simulink subsystem "Magnetometer"  (R2021a)
settings: Solver=VariableStepAuto  StartTime=0.0  StopTime=10.0  RelTol=1e-3
libraries: simulink x4, sharedtransform x1
settings Model: Creator=jmher  LastModifiedBy=jmher

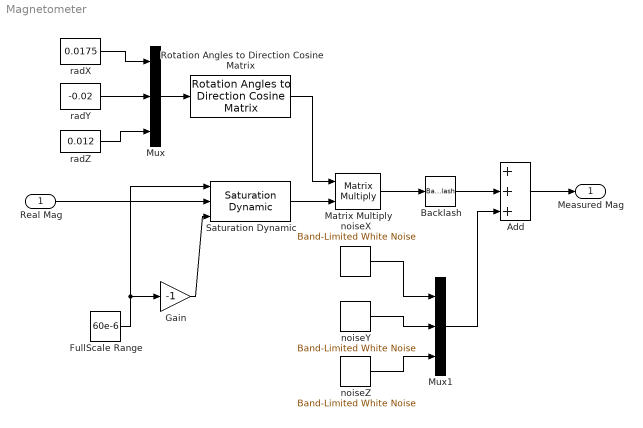
== system Magnetometer ==
  Real Mag : Inport
  Add : Sum  Inputs=+|+|+
  Backlash : Backlash  BacklashWidth=hyst  InputProcessing=Columns as channels (frame based)
  FullScale Range : Constant  Value=60e-6
  Gain : Gain  Gain=-1
  Matrix Multiply : Product  Multiplication=Matrix(*)
  Mux : Mux  Inputs=3
  Mux1 : Mux  Inputs=3
  Rotation Angles to Direction Cosine Matrix : sharedtransform/Rotation Angles to Direction Cosine Matrix  rotationOrder=ZYX  aMode=aMode
      settings: SourceProductBaseCode=AE,PW,DR,MT,UV,VE
  Saturation Dynamic : simulink/Discontinuities/Saturation Dynamic  OutMin=[]  OutMax=[]  OutDataTypeStr=Inherit: Same as second input  OutDataType=fixdt(1, 16)  OutScaling=2^-10  DoSatur=off
  noiseX : simulink/Sources/Band-Limited White Noise  Cov=noiseDens  Ts=0.1  seed=[47561]
  noiseY : simulink/Sources/Band-Limited White Noise  Cov=noiseDens  Ts=0.1  seed=[238641]
  noiseZ : simulink/Sources/Band-Limited White Noise  Cov=noiseDens  Ts=0.1  seed=[23341]
  radX : Constant  Value=0.0175
  radY : Constant  Value=-0.02
  radZ : Constant  Value=0.012
  Measured Mag : Outport
  wires:
  FullScale Range/1 -> Saturation Dynamic/1, Gain/1
  Gain/1 -> Saturation Dynamic/3
  Real Mag/1 -> Saturation Dynamic/2
  Mux/1 -> Rotation Angles to Direction Cosine Matrix/1
  radX/1 -> Mux/1
  radY/1 -> Mux/2
  radZ/1 -> Mux/3
  Rotation Angles to Direction Cosine Matrix/1 -> Matrix Multiply/1
  Matrix Multiply/1 -> Backlash/1
  Saturation Dynamic/1 -> Matrix Multiply/2
  noiseX/1 -> Mux1/1
  noiseY/1 -> Mux1/2
  noiseZ/1 -> Mux1/3
  Add/1 -> Measured Mag/1
  Backlash/1 -> Add/2
  Mux1/1 -> Add/3
